simulink model "Progetto4cSimulink"  (R2020b)
settings: Solver=VariableStepAuto  StartTime=0.0  StopTime=10.0  RelTol=1e-3
values from neighbouring files (symbols this model uses):
  A = [0 , 1; 0 , -(bb/(Mi*Ei*Ei+Ie))-(( (Ud*Mi*Ei*Ei)/(Mi*Ei*Ei+Ie) )*2*We) ]    [Progetto3a.m]    (also in Progetto4c.m = [0, 1; ((-gg*mm*ee)*cos(pi/2))/((mm*ee*ee+Ie)), -beta/(mm*ee; ProgettoGruppoAO.m; Progetto_Ada.m = [0, 1; ((-gg*mm*ee)*cos(pi/2))/((mm*ee*ee+Ie)), -beta/(mm*ee; Prova.m = [0, 1; 0, (bb/(Mi*Ei*Ei+Ie))-(( (Ud*Mi*Ei*Ei)/(Mi*Ei*Ei+Ie) )
  B = [0; 1/(Mi*Ei*Ei+Ie)]    [Progetto3a.m]    (also in Progetto4c.m = [0;1/(mm*ee*ee + Ie)]; ProgettoGruppoAO.m; Progetto_Ada.m = [0;1/(mm*ee*ee + Ie)]; Prova.m = [0, 1/(Mi*Ei*Ei+Ie)])
  beta = 0.3    [Progetto4c.m]    (also in Progetto_Ada.m)
  C = [0 , 1]    [Progetto3a.m]    (also in Progetto4c.m = [0, 1]; ProgettoGruppoAO.m; Progetto_Ada.m = [0, 1]; Prova.m = [0, 1])
  den_r = d_r{1}    [Progetto3a.m]    (also in Progetto4c.m; ProgettoGruppoAO.m; Progetto_Ada.m; Prova.m)
  num_r = n_r{1}    [Progetto3a.m]    (also in Progetto4c.m; ProgettoGruppoAO.m; Progetto_Ada.m; Prova.m)
  omega_n = 100    [Progetto3a.m]    (also in Progetto4c.m = 120; ProgettoGruppoAO.m; Progetto_Ada.m = 120; Prova.m)
  W = 5    [Progetto3a.m]    (also in Progetto4c.m = 4; ProgettoGruppoAO.m; Progetto_Ada.m = 4; Prova.m)
  x0 = [0,We]    [Progetto3a.m]    (also in Progetto4c.m = [0;0]; ProgettoGruppoAO.m = [teta_e,We]; Progetto_Ada.m = [0;0]; Prova.m = [0;0])
settings Model: Creator=MW  LastModifiedBy=39345

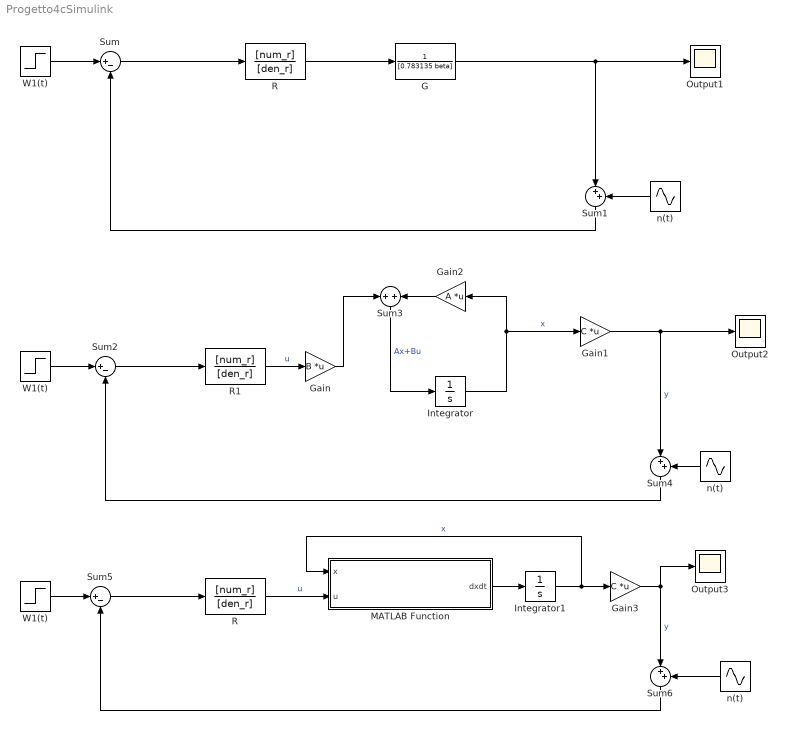
== system Progetto4cSimulink ==
  " n(t)  " : Sin  Amplitude=0.025  Frequency=omega_n  SampleTime=0  VectorParams1D=off
  G : TransferFcn  Denominator=[0.783135 beta]
  Gain : Gain  Gain=B  Multiplication=Matrix(K*u)
  Gain1 : Gain  Gain=C  Multiplication=Matrix(K*u)
  Gain2 : Gain  Gain=A  Multiplication=Matrix(K*u)
  Gain3 : Gain  Gain=C  Multiplication=Matrix(K*u)
  Integrator : Integrator  InitialCondition=x0
  Integrator1 : Integrator  InitialCondition=x0
  MATLAB Function : MATLAB Function  TreatAsAtomicUnit=on
  Output1 : Scope
  Output2 : Scope
  Output3 : Scope
  R : TransferFcn  Numerator=[num_r]  Denominator=[den_r]
  "R  " : TransferFcn  Numerator=[num_r]  Denominator=[den_r]
  R1 : TransferFcn  Numerator=[num_r]  Denominator=[den_r]
  Sum : Sum  Inputs=|+-
  Sum1 : Sum  Inputs=|++
  Sum2 : Sum  Inputs=|+-
  Sum3 : Sum
  Sum4 : Sum  Inputs=|++
  Sum5 : Sum  Inputs=|+-
  Sum6 : Sum  Inputs=|++
  W1(t) : Step  After=W  SampleTime=0
  "W1(t) " : Step  After=W  SampleTime=0
  "W1(t)  " : Step  After=W  SampleTime=0
  n(t) : Sin  Amplitude=0.025  Frequency=omega_n  SampleTime=0  VectorParams1D=off
  "n(t)  " : Sin  Amplitude=0.025  Frequency=omega_n  SampleTime=0  VectorParams1D=off
  wires:
  R/1 -> G/1
  G/1 -> Output1/1, Sum1/1
  W1(t)/1 -> Sum/1
  Sum/1 -> R/1
  Sum1/1 -> Sum/2
  n(t)/1 -> Sum1/2
  "W1(t) "/1 -> Sum2/1
  Sum2/1 -> R1/1
  R1/1 -> Gain/1  "u"
  Gain/1 -> Sum3/1
  Gain2/1 -> Sum3/2
  "n(t)  "/1 -> Sum4/2
  Gain1/1 -> Output2/1, Sum4/1  "y"
  Sum4/1 -> Sum2/2
  "W1(t)  "/1 -> Sum5/1
  Sum5/1 -> "R  "/1
  "R  "/1 -> MATLAB Function/2(u)  "u"
  MATLAB Function/1(dxdt) -> Integrator1/1
  Integrator1/1 -> MATLAB Function/1(x), Gain3/1  "x"
  Gain3/1 -> Output3/1, Sum6/1  "y"
  " n(t)  "/1 -> Sum6/2
  Sum6/1 -> Sum5/2
  Sum3/1 -> Integrator/1  "Ax+Bu"
  Integrator/1 -> Gain2/1, Gain1/1  "x"

== matlab function Progetto4cSimulink/MATLAB Function ==
  data: x input; u input; dxdt output
function dxdt = systemDynamic(x,u)
mm=0.15; %[kg] Mass
beta=0.3; %[N/m^2] Dynamic Friction coefficient
ee=0.47; % distanza asse rotazione
Ie = 0.75; %momento inerzia elica senza deformazione
gg=9.8065 %gravità
dx1dt=x(2);
dx2dt=(-beta*x(2)-(gg*mm*ee*sind(x(1))) + u)/(mm*ee*ee+Ie);
%dxdt = [dx1dt; dx2dt; dx3dt;...;dxndt];
dxdt = [dx1dt; dx2dt;];
